simulink model "Lab4"  (R2021b)
settings: Solver=FixedStepDiscrete  StartTime=0.0  StopTime=10.0  FixedStep=0.1  RelTol=1e-3  EnableMultiTasking=on
settings Model: Creator=Nerdan  LastModifiedBy=Nerdan
settings SolverCC: AlgebraicLoopSolver=TrustRegion  AutoInsertRateTranBlk=on
settings DataIOCC: LimitDataPoints=on
settings OptimizationCC: LifeSpan=inf
settings DebuggingCC: AllowSymbolicDim=off  SFUnexpectedBacktrackingDiag=warning  SFNoUnconditionalDefaultTransitionDiag=warning  SFExecutionAtInitializationDiag=none  ArithmeticOperatorsInVariantConditions=warning
settings SFSimCC: SimUseLocalCustomCode=off  CustomCodeUndefinedFunction=UseInterfaceOnly
settings RTWCC: RTWUseLocalCustomCode=off
settings CodeAppCC: StateflowObjectComments=on
settings GRTTargetCC: TargetLangStandard=C89/C90 (ANSI)
settings ConfigComp: CovMetricSettings=dw  CovSaveCumulativeToWorkspaceVar=on  CovSaveSingleToWorkspaceVar=on  CovExternalEMLEnable=off  CovSFcnEnable=off

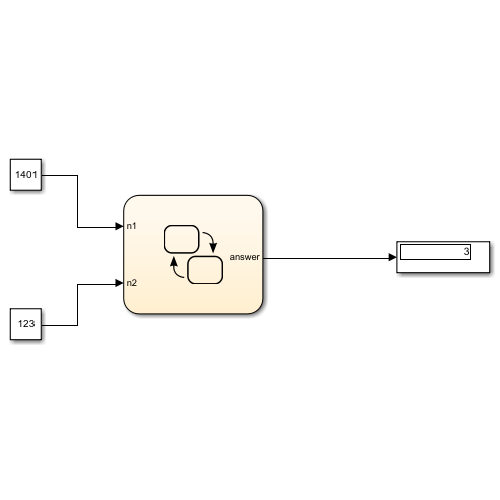
[thumbnail: Simulink's stored preview of the top-level diagram]
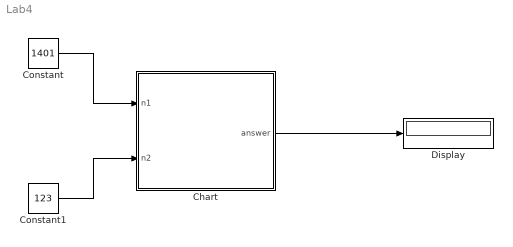
== system Lab4 ==
  Chart : Stateflow chart  TreatAsAtomicUnit=on
  Constant : Constant  Value=1401
  Constant1 : Constant  Value=123
  Display : Display
  wires:
  Chart/1(answer) -> Display/1
  Constant/1 -> Chart/1(n1)
  Constant1/1 -> Chart/2(n2)

== stateflow chart Lab4/Chart ==
  state answer
  (junction 9) -> (junction 6)
  (default) -> (junction 6) : {nn1=n1,nn2=n2}
  (junction 6) -> (junction 9) [order 1] : [nn1<nn2]{nn2=nn2-nn1}
  (junction 6) -> answer [order 3] : {answer=nn1}
  (junction 6) -> (junction 10) [order 2] : [nn2<nn1]{nn1=nn1-nn2}
  (junction 10) -> (junction 6)
  data: answer output; n1 input; n2 input; nn2 local; nn1 local
